simulink model "unity_feedback"  (R2022a)
settings: Solver=VariableStepAuto  StartTime=0.0  StopTime=30  RelTol=1e-3
libraries: simulink_extras x2
settings Model: Creator=pw705  LastModifiedBy=pw705

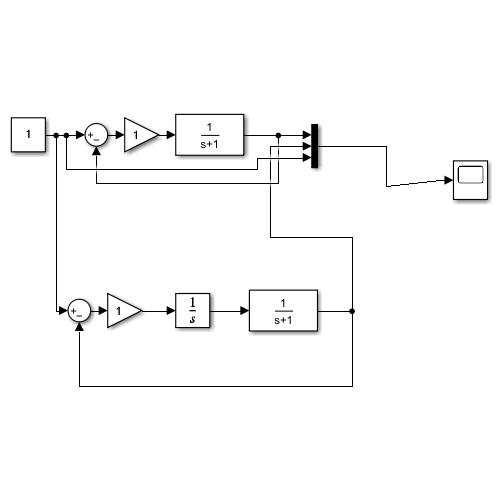
[thumbnail: Simulink's stored preview of the top-level diagram]
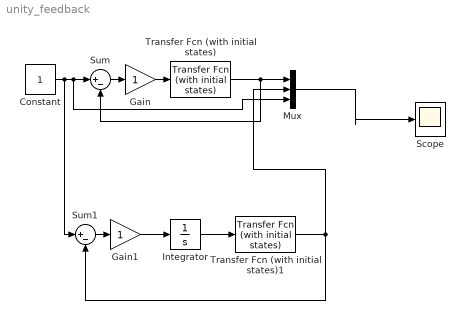
== system unity_feedback ==
  Constant : Constant
  Gain : Gain
  Gain1 : Gain
  Integrator : Integrator
  Mux : Mux  Inputs=3
  Scope : Scope
  Sum : Sum  Inputs=|+-
  Sum1 : Sum  Inputs=|+-
  Transfer Fcn (with initial states) : simulink_extras/Additional Linear/Transfer Fcn (with initial states)  N=[1]  D=[1 1]  X0=0
  Transfer Fcn (with initial states)1 : simulink_extras/Additional Linear/Transfer Fcn (with initial states)  N=[1]  D=[1 1]  X0=0
  wires:
  Sum/1 -> Gain/1
  Gain/1 -> Transfer Fcn (with initial states)/1
  Mux/1 -> Scope/1
  Transfer Fcn (with initial states)/1 -> Sum/2, Mux/1
  Gain1/1 -> Integrator/1
  Sum1/1 -> Gain1/1
  Constant/1 -> Sum1/1, Mux/3, Sum/1
  Transfer Fcn (with initial states)1/1 -> Mux/2, Sum1/2
  Integrator/1 -> Transfer Fcn (with initial states)1/1
